simulink model "sldemo_mdlref_fcncall"  (Simulink 7.6)
settings: Solver=FixedStepDiscrete  SolverMode=SingleTasking  StartTime=0.0  StopTime=15  FixedStep=0.005  RelTol=1e-3
libraries: simulink x1
settings Model: Creator=The MathWorks Inc.  ExtModeAutoUpdateStatusClock=off
settings DataIOCC: LimitDataPoints=off  SaveFormat=StructureWithTime  SignalLoggingName=logsOut
settings OptimizationCC: InlineParams=on  InlineInvariantSignals=on  InitFltsAndDblsToZero=on
settings DebuggingCC: SaveWithParameterizedLinksMsg=none  CheckExecutionContextPreStartOutputMsg=on  CheckExecutionContextRuntimeOutputMsg=on  SolverPrmCheckMsg=none  MultiTaskDSMMsg=warning  MultiTaskCondExecSysMsg=none  SigSpecEnsureSampleTimeMsg=none  StrictBusMsg=ErrorOnBusTreatedAsVector
settings HardwareCC: TargetHWDeviceType=32-bit Generic
settings ModelReferenceCC: UpdateModelReferenceTargets=IfOutOfDate  CheckModelReferenceTargetMessage=none
settings SFSimCC: SimParseCustomCode=off
settings RTWCC: GenerateReport=on  ProcessScript=grt_make_rtw_hook  LaunchReport=on  IncludeERTFirstTime=on
settings CodeAppCC: MaxIdLength=100
settings GRTTargetCC: TargetFcnLib=ansi_tfl_tmw.mat

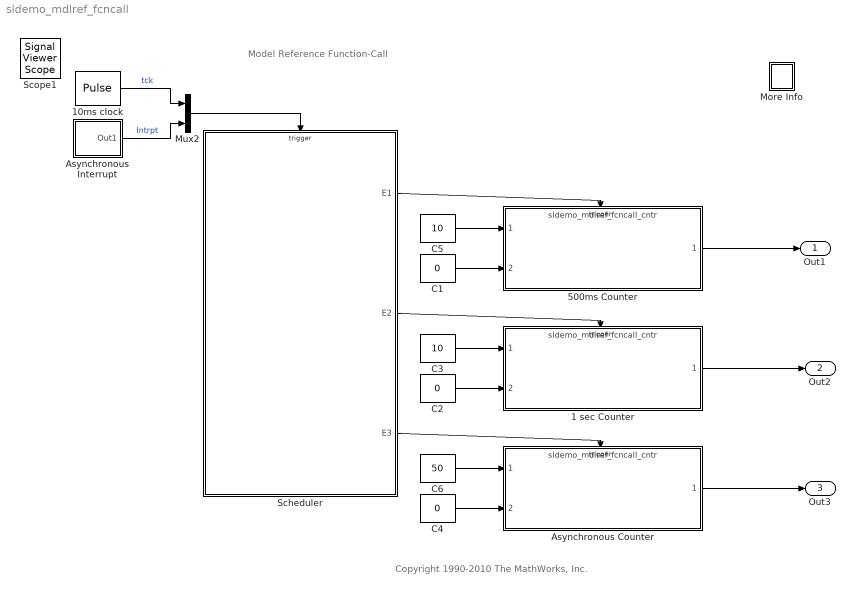
== system sldemo_mdlref_fcncall ==
  note: Model Reference Function-Call
  note: Copyright 1990-2010 The MathWorks, Inc.
  1 sec Counter : ModelReference  ModelNameDialog=sldemo_mdlref_fcncall_cntr  SimulationMode=Normal  ModelReferenceVersion=1.116  CopyOfModelName=sldemo_mdlref_fcncall_cntr  TriggerPortName=function  TriggerPortTriggerType=function-call  TriggerPortStatesWhenEnabling=held
  10ms clock : DiscretePulseGenerator  PulseType=Time based  Period=0.01  PulseWidth=50  SampleTime=0.005
  500ms Counter : ModelReference  ModelNameDialog=sldemo_mdlref_fcncall_cntr  SimulationMode=Normal  ModelReferenceVersion=1.116  CopyOfModelName=sldemo_mdlref_fcncall_cntr  TriggerPortName=function  TriggerPortTriggerType=function-call  TriggerPortStatesWhenEnabling=held
  "Asynchronous Interrupt " : Subsystem
      settings: RTWMemSecFuncInitTerm=Default  RTWMemSecFuncExecute=Default
  Asynchronous Counter : ModelReference  ModelNameDialog=sldemo_mdlref_fcncall_cntr  SimulationMode=Normal  ModelReferenceVersion=1.116  CopyOfModelName=sldemo_mdlref_fcncall_cntr  TriggerPortName=function  TriggerPortTriggerType=function-call  TriggerPortStatesWhenEnabling=held
  C1 : Constant  Value=0
  C2 : Constant  Value=0
  C3 : Constant  Value=10
  C4 : Constant  Value=0
  C5 : Constant  Value=10
  C6 : Constant  Value=50
  More Info : Subsystem
      settings: OpenFcn=showdemo(bdroot(gcb))
      mask Display: disp('?')
  Mux2 : Mux  Inputs=2
  Scheduler : Stateflow chart  TreatAsAtomicUnit=on
      settings: RTWMemSecFuncInitTerm=Default  RTWMemSecFuncExecute=Default
  Out1 : Outport
  Out2 : Outport  Port=2
  Out3 : Outport  Port=3
  Scope1 : SignalViewerScope  IOType=viewer  RefreshTime=0.035000
      settings: TimeRange=15  YMin=0  YMax=50
  wires:
  C5/1 -> 500ms Counter/1
  C1/1 -> 500ms Counter/2
  Scheduler/1(E1) -> 500ms Counter/Trigger
  Scheduler/2(E2) -> 1 sec Counter/Trigger
  C3/1 -> 1 sec Counter/1
  C2/1 -> 1 sec Counter/2
  C6/1 -> Asynchronous Counter/1
  C4/1 -> Asynchronous Counter/2
  Scheduler/3(E3) -> Asynchronous Counter/Trigger
  "Asynchronous Interrupt "/1(Out1) -> Mux2/2  "Intrpt"
  Asynchronous Counter/1 -> Out3/1
  500ms Counter/1 -> Out1/1
  1 sec Counter/1 -> Out2/1
  Mux2/1 -> Scheduler/Trigger
  10ms clock/1 -> Mux2/1  "tck"

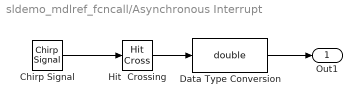
== system sldemo_mdlref_fcncall/Asynchronous Interrupt  ==
  Chirp Signal : simulink/Sources/Chirp Signal  SystemSampleTime=-1  f1=0.025  T=8  f2=5
  Data Type Conversion : DataTypeConversion  OutDataTypeStr=double
  Hit  Crossing : HitCross
  Out1 : Outport
  wires:
  Chirp Signal/1 -> Hit  Crossing/1
  Hit  Crossing/1 -> Data Type Conversion/1
  Data Type Conversion/1 -> Out1/1

== system sldemo_mdlref_fcncall/More Info ==
  note: Bus Block Demonstration
  note: This demonstration shows how signals may be grouped and ungrouped while
      | retaining their names.  In this demonstration, 5 signals are created and labelled
      | appropriately.  These signals are then mux'd together to create a bus of signals.
      | This bus of signals is then fed into the Bus Selector block.  Inside of the Bus
      | Selector block, the Pulse and Chirp signals are chosen to be output from the
      | original signal bus.
      |
      | It is possible to place a nest signal buses and then still retrieve the original signal
      | with its label.

== stateflow chart Scheduler ==
  note: This is a simple scheduler using
      | temporal logic and output events E1,E2
  state SynchronousScheduler [parallel]
    % 500ms rate
    on every(50,tck): send(E1);
    % 1sec rate
    on every(100,tck): send(E2);
    settings: executionOrder=2
  state AsynchronousScheduler [parallel]
    % Based on input Intrpt,
    % evaluated at clock base rate (10ms)
    settings: executionOrder=1
    AsynchronousScheduler -> (junction 7) : Intrpt{send(E3)}
  note: This is an asynchronous scheduler using
      | input event Intrpt, and output event E3
      | The asynchronous scheduler will be evaluated before
      | the synchronous scheduler.
  events: E1 output FUNCTION_CALL_EVENT; E2 output FUNCTION_CALL_EVENT; tck input RISING_EDGE_EVENT; E3 output FUNCTION_CALL_EVENT; Intrpt input RISING_EDGE_EVENT
